simulink model "SPEED_CONTROL_OF_BLDC_updated"  (R2023a)
settings: Solver=VariableStepAuto  StartTime=0.0  StopTime=0.5  RelTol=1e-3
libraries: hdlsllib x6, spsMosfetLib x6, spsControlledVoltageSourceLib x1, spsGroundLib x1, slpidlib x1, spsPermanentMagnetSynchronousMachineLib x1, spspowerguiLib x1
settings Model: Creator=sudib  LastModifiedBy=debjy

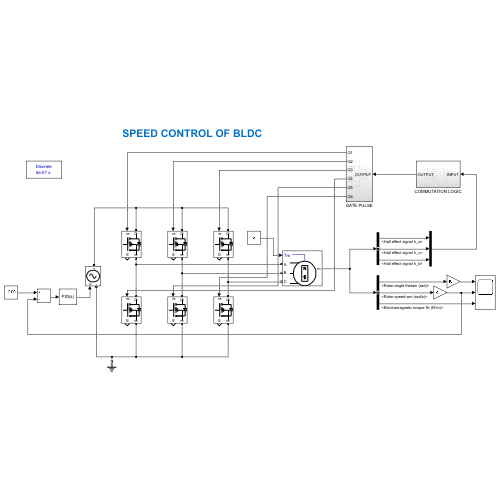
[thumbnail: Simulink's stored preview of the top-level diagram]
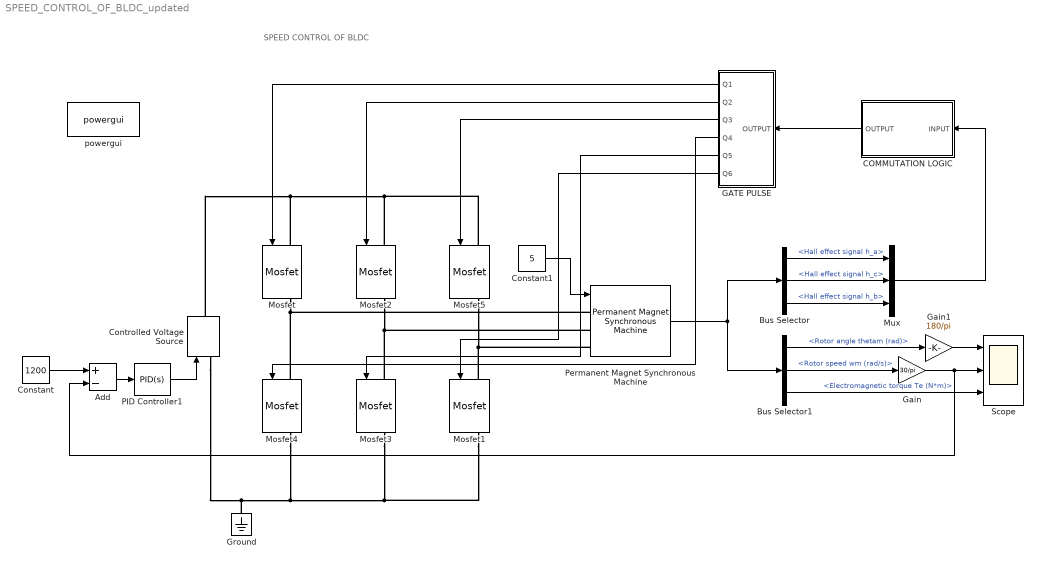
== system SPEED_CONTROL_OF_BLDC_updated ==
  note: SPEED CONTROL OF BLDC
  Add : Sum  Inputs=+-
  Bus Selector : BusSelector  OutputSignals=Hall effect signal h_a,Hall effect signal h_c,Hall effect signal h_b
  Bus Selector1 : BusSelector  OutputSignals=Rotor angle thetam (rad),Rotor speed wm (rad/s),Electromagnetic torque Te (N*m)
  COMMUTATION LOGIC : Subsystem
  Constant : Constant  Value=1200
  Constant1 : Constant  Value=5
  Controlled Voltage Source : spsControlledVoltageSourceLib/Controlled Voltage Source  Initialize=on  Source_Type=DC  Amplitude=160  Phase=0  Frequency=0  Measurements=None
  GATE PULSE : Subsystem
  Gain : Gain  Gain=30/pi
  Gain1 : Gain  Gain=180/pi
  Ground : spsGroundLib/Ground  LConnTagsString=a
  Mosfet{,1..5} (6 alike) : spsMosfetLib/Mosfet  Ron=0.1  Lon=0  Rd=0.01  Vfd=0  IC=0  Rs=1e5  Cs=inf  Measurements=on
  Mux : Mux  Inputs=3
  PID Controller1 : slpidlib/PID Controller  Controller=PID  Form=Parallel  TimeDomain=Continuous-time  UseExternalTs=off  SampleTime=-1  IntegratorMethod=Forward Euler  FilterMethod=Forward Euler  ControllerParametersSource=internal  P=0.01035  I=12.777  UseKiTs=off  D=12.564  N=0  UseFilter=on  TunerSelectOption=Transfer Function Based (PID Tuner App)  InitialConditionSource=internal  InitialConditionForIntegrator=0  InitialConditionForFilter=0  DifferentiatorICPrevScaledInput=0  ExternalReset=none  TrackingMode=off  Kt=1  LimitOutput=off  SatLimitsSource=internal  UpperSaturationLimit=inf  LowerSaturationLimit=-inf  LinearizeAsGain=on  AntiWindupMode=none  Kb=1  LimitIntegrator=off  UpperIntegratorSaturationLimit=inf  LowerIntegratorSaturationLimit=-inf  POutMin=[]  POutMax=[]  IOutMin=[]  IOutMax=[]  DOutMin=[]  DOutMax=[]  NOutMin=[]  NOutMax=[]  SumOutMin=[]  SumOutMax=[]  SaturationOutMin=[]  SaturationOutMax=[]  PParamMin=[]  PParamMax=[]  IParamMin=[]  IParamMax=[]  DParamMin=[]  DParamMax=[]  NParamMin=[]  NParamMax=[]  KbParamMin=[]  KbParamMax=[]  KtParamMin=[]  KtParamMax=[]  KbOutMin=[]  KbOutMax=[]  KtOutMin=[]  KtOutMax=[]  IntegratorOutMin=[]  IntegratorOutMax=[]  FilterOutMin=[]  FilterOutMax=[]  SumI1OutMin=[]  SumI1OutMax=[]  SumI2OutMin=[]  SumI2OutMax=[]  SumI3OutMin=[]  SumI3OutMax=[]  SumI4OutMin=[]  SumI4OutMax=[]  SumDOutMin=[]  SumDOutMax=[]  DifferentiatorOutMin=[]  DifferentiatorOutMax=[]  FilterDiffOutCoefMin=[]  FilterDiffOutCoefMax=[]  ReciprocalOutMin=[]  ReciprocalOutMax=[]  SumDenOutMin=[]  SumDenOutMax=[]  SumNumOutMin=[]  SumNumOutMax=[]  DivideOutMin=[]  DivideOutMax=[]  UdiffTsProdOutMin=[]  UdiffTsProdOutMax=[]  NTsProdOutMin=[]  NTsProdOutMax=[]  UintegralTsProdOutMin=[]  UintegralTsProdOutMax=[]  UngainTsProdOutMin=[]  UngainTsProdOutMax=[]  ClampingZeroOutDataTypeStr=Inherit: Inherit via back propagation  ClampingZeroOutMin=[]  ClampingZeroOutMax=[]  FilterDenConstantOutDataTypeStr=Inherit: Inherit via back propagation  FilterDenConstantOutMin=[]  FilterDenConstantOutMax=[]  PCopyOutDataTypeStr=Inherit: Inherit via back propagation  PCopyOutMin=[]  PCopyOutMax=[]  NCopyOutDataTypeStr=Inherit: Inherit via back propagation  NCopyOutMin=[]  NCopyOutMax=[]  IntegratorContinuousStateAttributes=''  IntegratorStateMustResolveToSignalObject=off  IntegratorRTWStateStorageClass=Auto  FilterContinuousStateAttributes=''  FilterStateMustResolveToSignalObject=off  FilterRTWStateStorageClass=Auto  ParallelPVariant=InternalParameters  IdealPVariant=Disabled  IVariant=InternalParameters  DVariant=InternalParameters  IntegratorVariant=Continuous  SatVariant=Disabled  AWVariant=Passthrough  PCopyVariant=Disabled  TRVariant=Disabled  FdbkBlocksVariant=Forward  IdealPFdbkVariant=Disabled  SatFdbkVariant=Disabled  DerivativeFilterVariant=ContFilter  NVariant=InternalParameters  NCopyVariant=Disabled  FilterICVariant=InternalICsFilter  IntegratorICVariant=InternalICs  ExternalResetVariant=Disabled  TRSumVariant=Passthrough  SumFdbkVariant=Disabled  SumVariant=Sum_PID  TsampFilterVariant=InternalTs  TsampNgainVariant=Passthrough  TsampIntegralVariant=Disabled_SignalSpec  ExternalSaturationOutDataTypeStr=Inherit: Same as second input
  Permanent Magnet Synchronous Machine : spsPermanentMagnetSynchronousMachineLib/Permanent Magnet Synchronous Machine  NbPhases=3  FluxDistribution=Trapezoidal  RotorType=Round  MechanicalLoad=Torque Tm  PresetModel=No  ShowDetailedParameters=on  MeasurementBus=off  Resistance=0.7  Inductance=2.7e-3  dqInductances=[8.5e-3,8.5e-3]  La=0.000395  MachineConstant=Flux linkage established by magnets (V.s)  Flux=0.1194  VoltageCst=100.0283  TorqueCst=0.9552  Flat=120  Mechanical=[0.0027 0.0004924 4 0]  PolePairs=4  InitialConditions=[0,0, 0,0]  InitialConditions5ph=[0 0 0 0 0 0]  RefAngle=90 degrees behind phase A axis (modified Park)  IterativeDiscreteModel=Trapezoidal non iterative  TsBlock=-1  TsPowergui=0
  Scope : Scope  NumInputPorts=3
  powergui : spspowerguiLib/powergui  Priority=1  SimulationMode=Discrete  SampleTime=50e-8  frequency=60  Iterations=50  frequencyindice=0  Pbase=100e6  ErrMax=1e-4  UnitsV=kV  UnitsW=MW  buscounter=0  FunctionMessages=off  echomessages=off  EnableUseOfTLC=off  CurrentSourceSwitches=off  DisableSnubberDevices=off  DisableRonSwitches=off  DisableVfSwitches=off  DisplayEquations=off  AutomaticDiscreteSolvers=off  SolverType=Tustin/Backward Euler (TBE)  Interpol=off  ExternalGateDelay=off  methode=off  Ts=100  x0status=blocks  SPID=on  SwTol=0  HookPort=off  NonlinearTolerance=1e-4  nMaxIteration=100  ContinueOnMaxIteration=off  RestoreLinks=warning  ResistiveCurrentMeasurement=off  Frange=[0:2:500]  Ylog=off  Xlog=on  ShowGrid=off  save=off  variable=ZData  structure=0  ZoomFFT=off  StartTime=0.0  cycles=1  DisplayStyle=1  fundamental=60  FreqAxis=off  MaxFrequency=1000  frequencyindicesteady=1  RmsSteady=1  display=off
  wires:
  Bus Selector1/2 -> Gain/1  "<Rotor speed wm (rad/s)>"
  Bus Selector1/1 -> Gain1/1  "<Rotor angle thetam (rad)>"
  Bus Selector1/3 -> Scope/3  "<Electromagnetic torque Te (N*m)>"
  Bus Selector/1 -> Mux/1  "<Hall effect signal h_a>"
  Constant/1 -> Add/1
  GATE PULSE/1(Q1) -> Mosfet/1
  Bus Selector/3 -> Mux/3  "<Hall effect signal h_b>"
  Permanent Magnet Synchronous Machine/1 -> Bus Selector1/1, Bus Selector/1
  Bus Selector/2 -> Mux/2  "<Hall effect signal h_c>"
  Mux/1 -> COMMUTATION LOGIC/1(INPUT)
  PID Controller1/1 -> Controlled Voltage Source/1
  Add/1 -> PID Controller1/1
  COMMUTATION LOGIC/1(OUTPUT) -> GATE PULSE/1(OUTPUT)
  Constant1/1 -> Permanent Magnet Synchronous Machine/1
  Gain/1 -> Add/2, Scope/2
  Gain1/1 -> Scope/1
  GATE PULSE/2(Q2) -> Mosfet2/1
  GATE PULSE/3(Q3) -> Mosfet5/1
  GATE PULSE/4(Q4) -> Mosfet4/1
  GATE PULSE/5(Q5) -> Mosfet3/1
  GATE PULSE/6(Q6) -> Mosfet1/1
  connections:
  Permanent Magnet Synchronous Machine/LConn1 -- Mosfet4/LConn1 -- Mosfet/RConn1
  Permanent Magnet Synchronous Machine/LConn2 -- Mosfet3/LConn1 -- Mosfet2/RConn1
  Controlled Voltage Source/LConn1 -- Mosfet1/RConn1 -- Mosfet3/RConn1 -- Mosfet4/RConn1 -- Ground/LConn1
  Controlled Voltage Source/RConn1 -- Mosfet/LConn1 -- Mosfet5/LConn1 -- Mosfet2/LConn1
  Permanent Magnet Synchronous Machine/LConn3 -- Mosfet1/LConn1 -- Mosfet5/RConn1

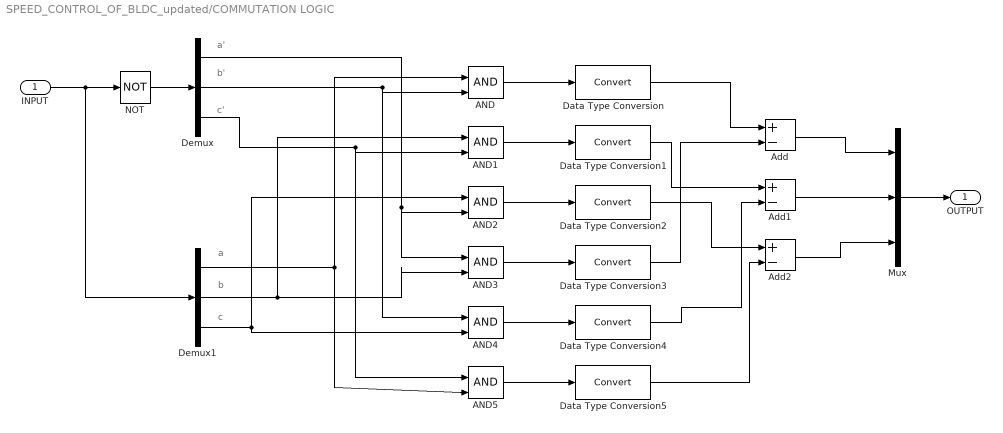
== system SPEED_CONTROL_OF_BLDC_updated/COMMUTATION LOGIC ==
  note: c
  note: a'
  note: b
  note: c'
  note: b'
  note: a
  INPUT : Inport
  AND{,1..5} (6 alike) : Logic  IconShape=distinctive  AllPortsSameDT=off  OutDataTypeStr=boolean
  Add : Sum  Inputs=+-
  Add1 : Sum  Inputs=+-
  Add2 : Sum  Inputs=+-
  Data Type Conversion{,1..5} (6 alike) : DataTypeConversion  SaturateOnIntegerOverflow=off  RndMeth=Floor
  Demux : Demux  Outputs=3
  Demux1 : Demux  Outputs=3
  Mux : Mux  Inputs=3
  NOT : Logic  Operator=NOT  IconShape=distinctive  AllPortsSameDT=off  OutDataTypeStr=boolean
  OUTPUT : Outport
  wires:
  Demux/1 -> AND3/1, AND2/2
  Demux1/3 -> AND4/2, AND2/1
  Demux/2 -> AND4/1, AND/2
  NOT/1 -> Demux/1
  Add1/1 -> Mux/2
  INPUT/1 -> Demux1/1, NOT/1
  Demux/3 -> AND5/1, AND1/2
  Demux1/2 -> AND1/1, AND3/2
  Add2/1 -> Mux/3
  Add/1 -> Mux/1
  Demux1/1 -> AND5/2, AND/1
  Mux/1 -> OUTPUT/1
  AND/1 -> Data Type Conversion/1
  AND5/1 -> Data Type Conversion5/1
  AND4/1 -> Data Type Conversion4/1
  AND3/1 -> Data Type Conversion3/1
  AND2/1 -> Data Type Conversion2/1
  AND1/1 -> Data Type Conversion1/1
  Data Type Conversion/1 -> Add/1
  Data Type Conversion5/1 -> Add2/2
  Data Type Conversion4/1 -> Add1/2
  Data Type Conversion3/1 -> Add/2
  Data Type Conversion2/1 -> Add2/1
  Data Type Conversion1/1 -> Add1/1

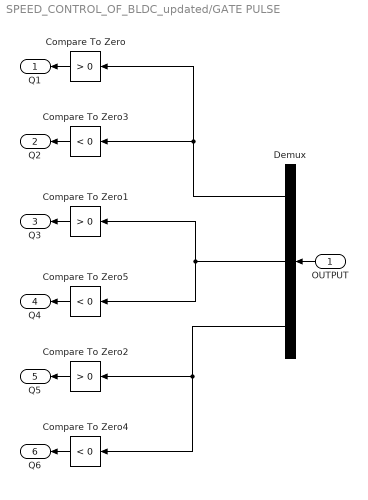
== system SPEED_CONTROL_OF_BLDC_updated/GATE PULSE ==
  OUTPUT : Inport
  Compare To Zero : hdlsllib/Logic and Bit Operations/Compare To Zero  relop=>  OutDataTypeStr=boolean
  Compare To Zero1 : hdlsllib/Logic and Bit Operations/Compare To Zero  relop=>  OutDataTypeStr=boolean
  Compare To Zero2 : hdlsllib/Logic and Bit Operations/Compare To Zero  relop=>  OutDataTypeStr=boolean
  Compare To Zero3 : hdlsllib/Logic and Bit Operations/Compare To Zero  relop=<  OutDataTypeStr=boolean
  Compare To Zero4 : hdlsllib/Logic and Bit Operations/Compare To Zero  relop=<  OutDataTypeStr=boolean
  Compare To Zero5 : hdlsllib/Logic and Bit Operations/Compare To Zero  relop=<  OutDataTypeStr=boolean
  Demux : Demux  Outputs=3
  Q1 : Outport
  Q2 : Outport  Port=2
  Q3 : Outport  Port=3
  Q4 : Outport  Port=4
  Q5 : Outport  Port=5
  Q6 : Outport  Port=6
  wires:
  Compare To Zero/1 -> Q1/1
  Demux/3 -> Compare To Zero4/1, Compare To Zero2/1
  Demux/2 -> Compare To Zero1/1, Compare To Zero5/1
  Compare To Zero4/1 -> Q6/1
  Compare To Zero3/1 -> Q2/1
  Demux/1 -> Compare To Zero3/1, Compare To Zero/1
  OUTPUT/1 -> Demux/1
  Compare To Zero2/1 -> Q5/1
  Compare To Zero1/1 -> Q3/1
  Compare To Zero5/1 -> Q4/1
